simulink model "mdl2"  (R2013b)
settings: Solver=ode1  StartTime=0.0  StopTime=tSim  FixedStep=h  RelTol=1e-3
settings Model: Creator=JAR  LastModifiedBy=JAR

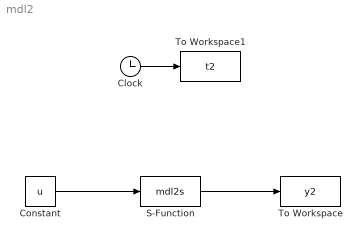
== system mdl2 ==
  Clock : Clock
  Constant : Constant  Value=u
  S-Function : S-Function  FunctionName=mdl2s  Parameters=y0  EnableBusSupport=off
  To Workspace : ToWorkspace  VariableName=y2  SampleTime=-1
  To Workspace1 : ToWorkspace  VariableName=t2  SampleTime=-1
  wires:
  Clock/1 -> To Workspace1/1
  Constant/1 -> S-Function/1
  S-Function/1 -> To Workspace/1
